simulink model "MotorEstimation"  (R2023b)
settings: Solver=VariableStepAuto  StartTime=0.0  StopTime=30  MaxStep=0.01  RelTol=1e-3
InitFcn:
  | JointParameters
values from neighbouring files (symbols this model uses):
  a = 0    [JointParameters.m]
  b = 1    [JointParameters.m]
  B_l = 0.05    [JointParameters.m]
  B_u = 0    [JointParameters.m]
  c = 1    [JointParameters.m]
  Current_Thrust = 50    [JointParameters.m]
  g = 9.81    [JointParameters.m]
  Input_Power = 1    [JointParameters.m]
  J_l = 0.065561919    [JointParameters.m]
  J_u = 0.045179    [JointParameters.m]
  k = 0.3    [JointParameters.m]
  L_cg_l = 0.101389    [JointParameters.m]
  L_cg_u = 0.066582    [JointParameters.m]
  L_l = 0.2225794    [JointParameters.m]
  L_u = 0.227293    [JointParameters.m]
  mass_l = 2.292    [JointParameters.m]
  mass_u = 1.821    [JointParameters.m]
libraries: simulink x1
settings Model: Creator=user  LastModifiedBy=user

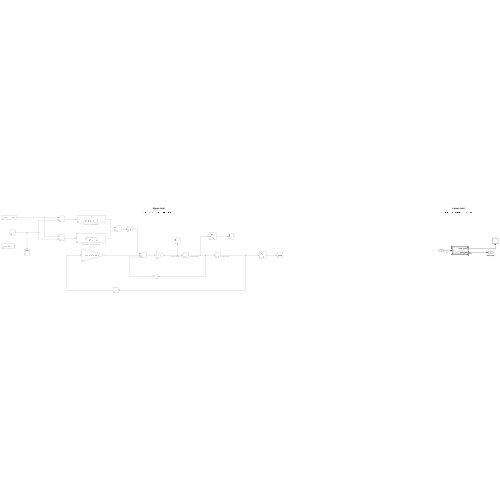
[thumbnail: Simulink's stored preview of the top-level diagram]
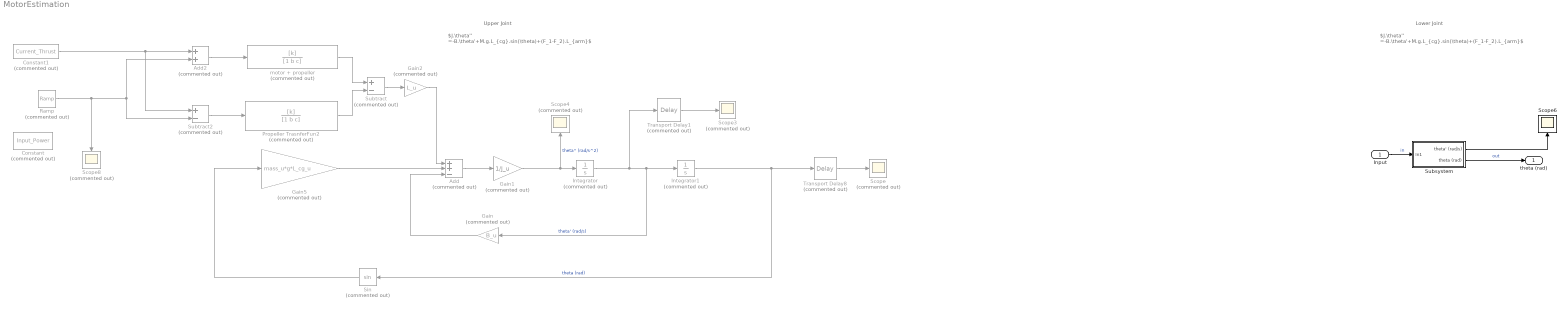
== system MotorEstimation ==
  note: $J.\theta'' =-B.\theta'+M.g.L_{cg}.sin(\theta)+(F_1-F_2).L_{arm}$
  note: Upper Joint
  note: $J.\theta'' =-B.\theta'+M.g.L_{cg}.sin(\theta)+(F_1-F_2).L_{arm}$
  note: Lower Joint
  Input : Inport
  Add : Sum  Commented=on  Inputs=++-
  Add2 : Sum  Commented=on
  Constant : Constant  Commented=on  Value=Input_Power
  Constant1 : Constant  Commented=on  Value=Current_Thrust
  Gain : Gain  Commented=on  Gain=B_u
  Gain1 : Gain  Commented=on  Gain=1/J_u
  Gain2 : Gain  Commented=on  Gain=L_u
  Gain5 : Gain  Commented=on  Gain=mass_u*g*L_cg_u
  Integrator : Integrator  Commented=on
  Integrator1 : Integrator  Commented=on  InitialCondition=-15*pi/180  LimitOutput=on  UpperSaturationLimit=15*pi/180  LowerSaturationLimit=-15*pi/180
  Propeller TrasnferFun2 : TransferFcn  Commented=on  Numerator=[k]  Denominator=[1 b c]
  Ramp : simulink/Sources/Ramp  Commented=on  slope=0.1  start=0  InitialOutput=0
  Scope{,3..4,8} (4 alike) : Scope  Commented=on
  Scope6 : Scope
  Sin : Trigonometry  Commented=on
  Subsystem : Subsystem
  Subtract : Sum  Commented=on  Inputs=+-
  Subtract2 : Sum  Commented=on  Inputs=+-
  Transport Delay1 : TransportDelay  Commented=on  DelayTime=0.0225
  Transport Delay8 : TransportDelay  Commented=on  DelayTime=0.0225
  motor + propeller : TransferFcn  Commented=on  Numerator=[k]  Denominator=[1 b c]
  theta (rad) : Outport
  wires:
  Gain1/1 -> Scope4/1, Integrator/1  "theta'' (rad/s^2)"
  Integrator/1 -> Transport Delay1/1, Gain/1, Integrator1/1  "theta' (rad/s)"
  Integrator1/1 -> Sin/1, Transport Delay8/1  "theta (rad)"
  motor + propeller/1 -> Subtract/1
  Propeller TrasnferFun2/1 -> Subtract/2
  Subtract/1 -> Gain2/1
  Sin/1 -> Gain5/1
  Gain5/1 -> Add/2
  Gain/1 -> Add/3
  Add/1 -> Gain1/1
  Gain2/1 -> Add/1
  Subtract2/1 -> Propeller TrasnferFun2/1
  Add2/1 -> motor + propeller/1
  Constant1/1 -> Subtract2/1, Add2/1
  Ramp/1 -> Add2/2, Subtract2/2, Scope8/1
  Transport Delay8/1 -> Scope/1
  Transport Delay1/1 -> Scope3/1
  Input/1 -> Subsystem/1(In1)  "in"
  Subsystem/1(theta' (rad/s)) -> Scope6/1
  Subsystem/2(theta (rad)) -> theta (rad)/1  "out"

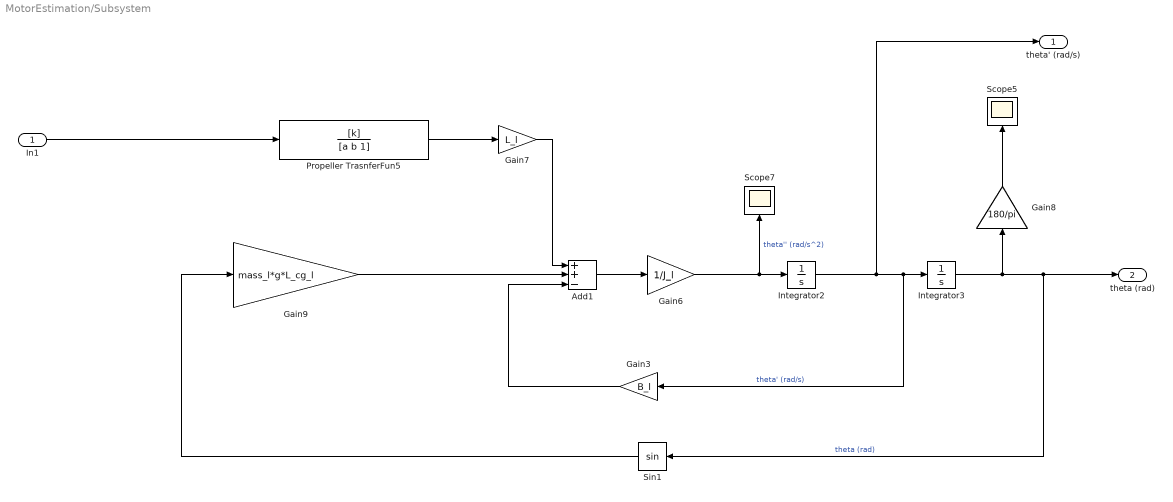
== system MotorEstimation/Subsystem ==
  In1 : Inport
  Add1 : Sum  Inputs=++-
  Gain3 : Gain  Gain=B_l
  Gain6 : Gain  Gain=1/J_l
  Gain7 : Gain  Gain=L_l
  Gain8 : Gain  Gain=180/pi
  Gain9 : Gain  Gain=mass_l*g*L_cg_l
  Integrator2 : Integrator
  Integrator3 : Integrator  InitialCondition=-0.33  LimitOutput=on  UpperSaturationLimit=0.4  LowerSaturationLimit=-0.33
  Propeller TrasnferFun5 : TransferFcn  Numerator=[k]  Denominator=[a b 1]
  Scope5 : Scope
  Scope7 : Scope
  Sin1 : Trigonometry
  theta' (rad/s) : Outport
  theta (rad) : Outport  Port=2
  wires:
  Gain3/1 -> Add1/3
  Integrator3/1 -> Gain8/1, theta (rad)/1, Sin1/1  "theta (rad)"
  Sin1/1 -> Gain9/1
  Propeller TrasnferFun5/1 -> Gain7/1
  Add1/1 -> Gain6/1
  Gain7/1 -> Add1/1
  Gain8/1 -> Scope5/1
  Gain9/1 -> Add1/2
  Integrator2/1 -> theta' (rad/s)/1, Integrator3/1, Gain3/1  "theta' (rad/s)"
  Gain6/1 -> Integrator2/1, Scope7/1  "theta'' (rad/s^2)"
  In1/1 -> Propeller TrasnferFun5/1
